simulink model "PT1_IM_KM"  (R2016a)
settings: Solver=FixedStepAuto  StartTime=0.0  StopTime=deltaT*(size(time,1)-1)  FixedStep=0.00001  RelTol=1e-3
values from neighbouring files (symbols this model uses):
  deltaT = M5_deltaT    [A1_Versuch1_Auswertung1.m]    (also in A2_Versuch1_Auswertung1.m; A2_Versuch1_Auswertung2.m; BestimmungCR_Holzbau.m)
  strom = M5_I_M    [A1_Versuch1_Auswertung1.m]    (also in A2_Versuch1_Auswertung1.m; A2_Versuch1_Auswertung2.m; BestimmungCR_Holzbau.m)
settings Model: Creator=ich  LastModifiedBy=ich

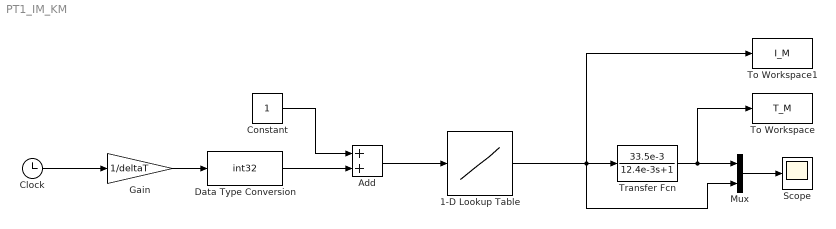
== system PT1_IM_KM ==
  1-D Lookup Table : Lookup_n-D  NumberOfTableDimensions=1  BreakpointsSpecification=Even spacing  BreakpointsForDimension1=[-5:5]  Table=strom  InternalRulePriority=Speed  RndMeth=Simplest  InputSameDT=on
  Add : Sum
  Clock : Clock
  Constant : Constant
  Data Type Conversion : DataTypeConversion  OutDataTypeStr=int32
  Gain : Gain  Gain=1/deltaT
  Mux : Mux  Inputs=2
  Scope : Scope
  To Workspace : ToWorkspace  VariableName=T_M  SampleTime=-1
  To Workspace1 : ToWorkspace  VariableName=I_M  SampleTime=-1
  Transfer Fcn : TransferFcn  Numerator=[33.5e-3]  Denominator=[12.4e-3 1]
  wires:
  1-D Lookup Table/1 -> To Workspace1/1, Mux/2, Transfer Fcn/1
  Clock/1 -> Gain/1
  Gain/1 -> Data Type Conversion/1
  Constant/1 -> Add/1
  Add/1 -> 1-D Lookup Table/1
  Data Type Conversion/1 -> Add/2
  Transfer Fcn/1 -> To Workspace/1, Mux/1
  Mux/1 -> Scope/1
